simulink model "DP2"  (R2022b)
settings: Solver=VariableStepAuto  StartTime=0.0  StopTime=3  RelTol=1e-3
values from neighbouring files (symbols this model uses):
  K_lqr = [   412.01  -1.93   1.32  307.69  -0.01   0.00  -94.28  -0.00  -0.00 ... (first row only)    [Matrices.m]
settings Model: Creator=darcyschofield  LastModifiedBy=darcyschofield

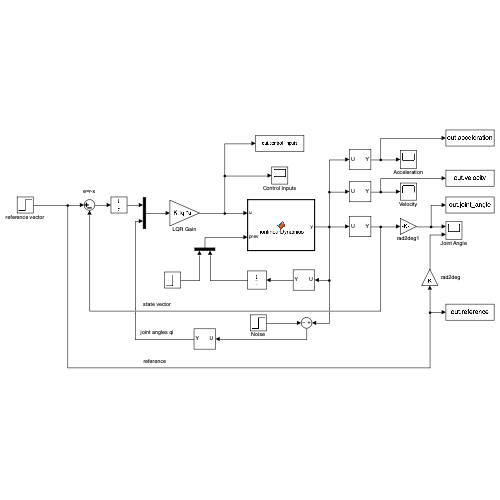
[thumbnail: Simulink's stored preview of the top-level diagram]
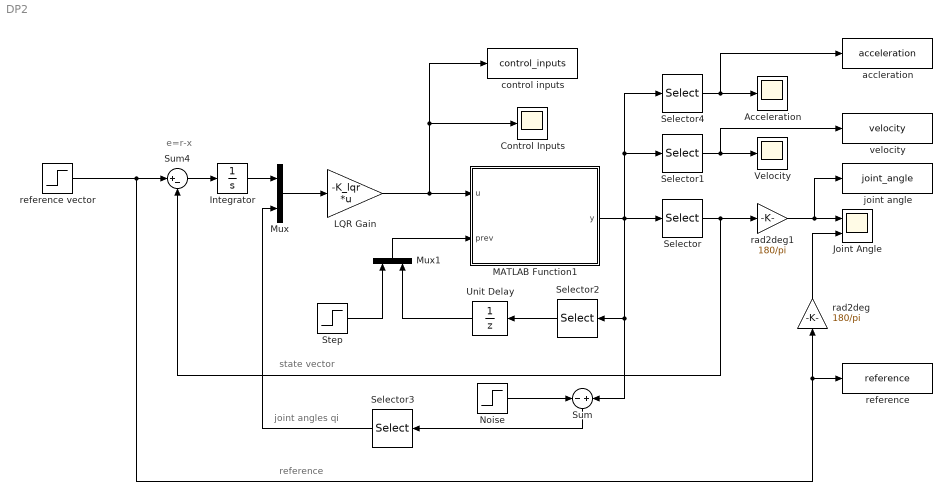
== system DP2 ==
  note: e=r-x
  note: joint angles qi
  note: reference
  note: state vector
  Acceleration : Scope
  Control Inputs : Scope
  Integrator : Integrator
  Joint Angle : Scope  NumInputPorts=2
  LQR Gain : Gain  Gain=-K_lqr  Multiplication=Matrix(K*u)  SaturateOnIntegerOverflow=on  OutDataTypeStr=Inherit: Same as input  ParamDataTypeStr=Inherit: Same as input
  MATLAB Function1 : MATLAB Function  TreatAsAtomicUnit=on
  Mux : Mux  Inputs=2
  Mux1 : Mux  Inputs=2
  Noise : Step  Time=0  After=0  SampleTime=0
  Selector : Selector  InputPortWidth=9  IndexOptions=Index vector (dialog)  Indices=[1 2 3]  OutputSizes=1
  Selector1 : Selector  InputPortWidth=9  IndexOptions=Index vector (dialog)  Indices=[4 5 6]  OutputSizes=1
  Selector2 : Selector  InputPortWidth=9  IndexOptions=Index vector (dialog)  Indices=[7 8 9]  OutputSizes=1
  Selector3 : Selector  InputPortWidth=9  IndexOptions=Index vector (dialog)  Indices=[1 2 3 4 5 6]  OutputSizes=1
  Selector4 : Selector  InputPortWidth=9  IndexOptions=Index vector (dialog)  Indices=[7 8 9]  OutputSizes=1
  Step : Step  Time=0  After=[0; 0; 0; 0; 0; 0]  SampleTime=0
  Sum : Sum  Inputs=-+
  Sum4 : Sum  Inputs=|+-  InputSameDT=on  SaturateOnIntegerOverflow=on  OutDataTypeStr=Inherit: Same as first input
  Unit Delay : UnitDelay  InitialCondition=[0; 0; 0]  SampleTime=-1  HasFrameUpgradeWarning=on
  Velocity : Scope
  accleration : ToWorkspace  VariableName=acceleration  SaveFormat=Timeseries  SampleTime=-1
  control inputs : ToWorkspace  VariableName=control_inputs  SaveFormat=Timeseries  SampleTime=-1
  joint angle : ToWorkspace  VariableName=joint_angle  SaveFormat=Timeseries  SampleTime=-1
  rad2deg : Gain  Gain=180/pi
  rad2deg1 : Gain  Gain=180/pi
  reference : ToWorkspace  VariableName=reference  SaveFormat=Timeseries  SampleTime=-1
  reference vector : Step  Time=0  Before=[0; 0; 0]  After=[1.75; 1.13; 2.18]  SampleTime=0
  velocity : ToWorkspace  VariableName=velocity  SaveFormat=Timeseries  SampleTime=-1
  wires:
  reference vector/1 -> rad2deg/1, reference/1, Sum4/1
  Selector/1 -> rad2deg1/1, Sum4/2
  Sum4/1 -> Integrator/1
  Integrator/1 -> Mux/1
  Selector3/1 -> Mux/2
  MATLAB Function1/1(y) -> Selector4/1, Selector1/1, Selector/1, Sum/2, Selector2/1
  Selector4/1 -> Acceleration/1, accleration/1
  Selector1/1 -> Velocity/1, velocity/1
  LQR Gain/1 -> Control Inputs/1, control inputs/1, MATLAB Function1/1(u)
  Unit Delay/1 -> Mux1/2
  Selector2/1 -> Unit Delay/1
  Step/1 -> Mux1/1
  Mux1/1 -> MATLAB Function1/2(prev)
  Mux/1 -> LQR Gain/1
  Sum/1 -> Selector3/1
  Noise/1 -> Sum/1
  rad2deg/1 -> Joint Angle/2
  rad2deg1/1 -> joint angle/1, Joint Angle/1

== matlab function DP2/MATLAB Function1 ==
  data: u input; y output; prev input
function y = nonlinearDynamics(u, prev)
% Vectorized discrete dynamics for a 3-link planar robot leg

% x_prev: 6x1 state vector = [q1; q2; q3; dq1; dq2; dq3]
% u_prev: 3x1 torque vector = [tau1; tau2; tau3]
% ddq_prev: 3x1 vector of previous accelerations
% dt: scalar time step

% Unpack inputs
q = prev(1:3);
dq = prev(4:6);
ddq_prev = prev(7:9);

tau = u;

q1 = q(1); q2 = q(2); q3 = q(3);
dq1 = dq(1); dq2 = dq(2); dq3 = dq(3);
tau1 = tau(1); tau2 = tau(2); tau3 = tau(3);
ddq1_prev = ddq_prev(1); ddq2_prev = ddq_prev(2); ddq3_prev = ddq_prev(3);

% Damping coeffs
b1 = 0.7;
b2 = 0.7;
b3 = 0.7;


ddq1 = (-5000000.0*b1*dq1 - 325845.0*ddq2_prev*cos(q2 + q3) - 2983860.0*ddq2_prev*cos(q2) - 637208.0*ddq2_prev*cos(q3) - 2092085.0*ddq2_prev...
        - 325845.0*ddq3_prev*cos(q2 + q3) - 318604.0*ddq3_prev*cos(q3) - 94133.0*ddq3_prev + 651690.0*dq1*dq2*sin(q2 + q3)...
        + 5967720.0*dq1*dq2*sin(q2) + 651690.0*dq1*dq3*sin(q2 + q3) + 637208.0*dq1*dq3*sin(q3) + 325845.0*dq2^2*sin(q2 + q3)...
        + 2983860.0*dq2^2*sin(q2) + 651690.0*dq2*dq3*sin(q2 + q3) + 637208.0*dq2*dq3*sin(q3) + 325845.0*dq3^2*sin(q2 + q3)...
        + 318604.0*dq3^2*sin(q3) + 5000000.0*tau1 + 65048148.0*cos(q1 + q2) + 7103421.0*cos(q1 + q2 + q3)...
        + 201168765.0*cos(q1))/(651690.0*cos(q2 + q3) + 5967720.0*cos(q2) + 637208.0*cos(q3) + 9193760.0);

ddq2 = (-5000000.0*b2*dq2 - 325845.0*ddq1_prev*cos(q2 + q3) - 2983860.0*ddq1_prev*cos(q2) - 637208.0*ddq1_prev*cos(q3) - 2092085.0*ddq1_prev...
        - 318604.0*ddq3_prev*cos(q3) - 94133.0*ddq3_prev - 325845.0*dq1^2*sin(q2 + q3) - 2983860.0*dq1^2*sin(q2)... 
        + 637208.0*dq1*dq3*sin(q3) + 637208.0*dq2*dq3*sin(q3) + 318604.0*dq3^2*sin(q3) + 5000000.0*tau2...
        + 65048148.0*cos(q1 + q2) + 7103421.0*cos(q1 + q2 + q3))/(637208.0*cos(q3) + 2092085.0);

ddq3 = -53.1163353977882*b3*dq3 - 3.46153846153846*ddq1_prev*cos(q2 + q3) - 3.38461538461538*ddq1_prev*cos(q3) - ddq1_prev... 
        - 3.38461538461538*ddq2_prev*cos(q3) - ddq2_prev - 3.46153846153846*dq1^2*sin(q2 + q3) - 3.38461538461538*dq1^2*sin(q3)... 
        - 6.76923076923077*dq1*dq2*sin(q3) - 3.38461538461538*dq2^2*sin(q3) + 53.1163353977882*tau3 + 75.4615384615385*cos(q1 + q2 + q3);

ddq = [ddq1; ddq2; ddq3];

% --- Discrete integration ---
dt = 0.2;
dq_next = dq + dt * ddq;
q_next  = q  + dt * dq_next;

y = [q_next; dq_next; ddq];

end
